simulink model "temperature"  (R2022b)
settings: Solver=VariableStepAuto  StartTime=0.0  StopTime=10.0  RelTol=1e-3
settings Model: Creator=Brigosha_Guest  LastModifiedBy=Brigosha_Guest

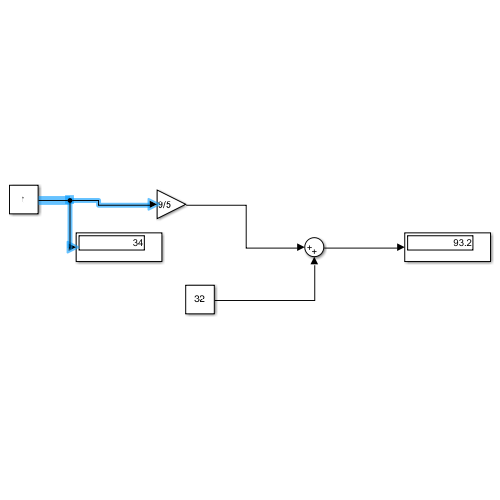
[thumbnail: Simulink's stored preview of the top-level diagram]
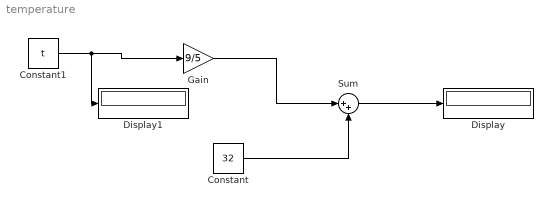
== system temperature ==
  Constant : Constant  Value=32
  Constant1 : Constant  Value=t
  Display : Display
  Display1 : Display
  Gain : Gain  Gain=9/5
  Sum : Sum  Inputs=|++
  wires:
  Gain/1 -> Sum/1
  Constant/1 -> Sum/2
  Constant1/1 -> Display1/1, Gain/1
  Sum/1 -> Display/1
